simulink model "ESD_Poject_Portable_solar_PV"  (R2024a)
settings: Solver=ode23t  StartTime=0.0  StopTime=5  RelTol=1e-3
undefined symbols (not defined in the file or in its folder): Ion, Lithium
libraries: spsSeriesRLCBranchLib x10, spsCurrentMeasurementLib x4, spsVoltageMeasurementLib x3, spsMosfetLib x2, spsIGBTDiodeLib x2, spsBatteryLib x1, spsDiodeLib x1, spsIGBTLib x1, slpidlib x1, spsPVArrayLib x1, eePwmGenerator x1, spsPWMGeneratorDCDCLib x1
settings Model: Creator=vihan  LastModifiedBy=vihan

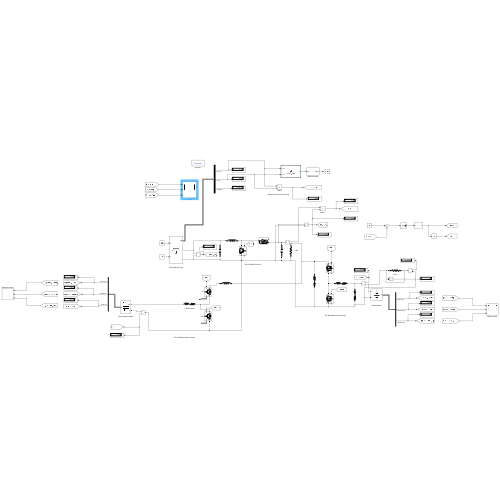
[thumbnail: Simulink's stored preview of the top-level diagram]
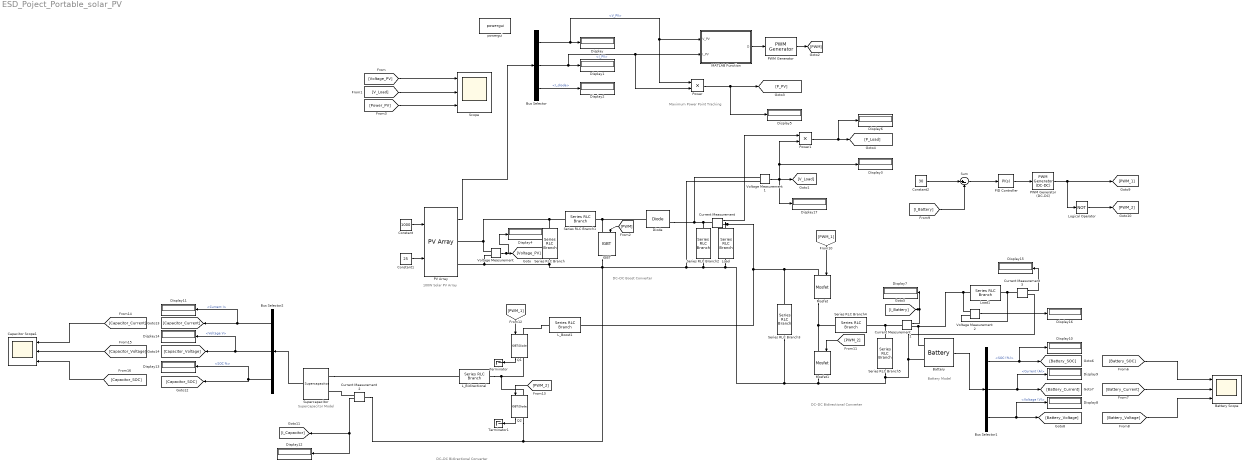
== system ESD_Poject_Portable_solar_PV ==
  note: Supercapacitor Model
  note: Battery Model
  note: DC–DC Bidirectional Converter
  note: Maximum Power Point Tracking
  note: DC–DC Boost Converter
  note: 100W Solar PV Array
  note: DC–DC Bidirectional Converter
  Battery : spsBatteryLib/Battery  BatType=Lithium-Ion  ShowTempParam=off  ThermalPreset=no  ShowAgeParam=off  NomV=7.2  NomQ=5.4  SOC=100  Batt_Tr=30  PresetModel=on  MaxQ=5.4  MinV=5.4  FullV=8.3807  Dis_rate=2.3478  R=0.013333  Normal_OP=4.8835  expZone="[7.7788      0.2653]"  current=[6.5 13 32.5]  Units=Time  Tci=20  NomT=20  T2=-30  MaxQ2=4.8  FullV2=7.1  Normal_OP2=5.655  expZone2="[6.58           1]"  Rca=0.6  ti=2000  Dp=0  Neq0=0  Tsim=1e6  Ta1=25  Qeol=5.4*0.9  Reol=0.013333*1.2  Char_age=[2.3478, 3]  Dis_age=[2.3478, 10]  N1=1500  N2=10500  N3=1000  N4=1400  Ta2=45  N5=950
  Battery Scope : Scope  NumInputPorts=3
  Bus Selector : BusSelector  OutputSignals=V_PV,I_PV,I_diode
  Bus Selector1 : BusSelector  OutputSignals=SOC (%),Current (A),Voltage (V)
  Bus Selector2 : BusSelector  OutputSignals=Current I,Voltage V,SOC %
  Capacitor Scope1 : Scope  NumInputPorts=3
  Constant : Constant  Value=1000
  Constant1 : Constant  Value=25
  Constant2 : Constant  Value=30
  Current Measurement{,1..3} (4 alike) : spsCurrentMeasurementLib/Current Measurement  PhasorSimulation=off  OutputType=Complex  PSBequivalent=0
  Diode : spsDiodeLib/Diode  Ron=0.001  Lon=0  Vf=0.8  IC=0  UseSnubber=0  Rs=500  Cs=250e-9  Measurements=on
  Display{,1..17} (18 alike) : Display
  IGBT : spsIGBTLib/IGBT  Ron=0.001  Lon=0  Vf=1  Tf=1e-6  Tt=2e-6  IC=0  Rs=1e5  Cs=inf  Measurements=on
  L_Bidirectional : spsSeriesRLCBranchLib/Series RLC Branch  LConnTagsString=__new0  RConnTagsString=__new0  BranchType=RL  Resistance=0.05  Inductance=0.355e-3  SetiL0=off  InitialCurrent=0  Capacitance=1e-6  Setx0=off  InitialVoltage=0  Measurements=None
  L_Boost1 : spsSeriesRLCBranchLib/Series RLC Branch  LConnTagsString=__new0  RConnTagsString=__new0  BranchType=L  Resistance=0.05  Inductance=1.5e-3  SetiL0=off  InitialCurrent=0  Capacitance=1e-6  Setx0=off  InitialVoltage=0  Measurements=None
  Load : spsSeriesRLCBranchLib/Series RLC Branch  LConnTagsString=__new0  RConnTagsString=__new0  BranchType=R  Resistance=50  Inductance=1e-3  SetiL0=off  InitialCurrent=0  Capacitance=3000e-6  Setx0=on  InitialVoltage=0  Measurements=None
  Load1 : spsSeriesRLCBranchLib/Series RLC Branch  LConnTagsString=__new0  RConnTagsString=__new0  BranchType=R  Resistance=500000  Inductance=1e-3  SetiL0=off  InitialCurrent=0  Capacitance=3000e-6  Setx0=on  InitialVoltage=0  Measurements=None
  Logical Operator : Logic  Operator=NOT  AllPortsSameDT=off  OutDataTypeStr=boolean
  MATLAB Function : MATLAB Function  TreatAsAtomicUnit=on
  Mosfet : spsMosfetLib/Mosfet  Ron=0.1  Lon=0  Rd=0.01  Vfd=0  IC=0  Rs=1e5  Cs=inf  Measurements=on
  Mosfet1 : spsMosfetLib/Mosfet  Ron=0.1  Lon=0  Rd=0.01  Vfd=0  IC=0  Rs=1e5  Cs=inf  Measurements=on
  PID Controller : slpidlib/PID Controller  Controller=PI  Form=Parallel  TimeDomain=Continuous-time  UseExternalTs=off  SampleTime=-1  IntegratorMethod=Forward Euler  FilterMethod=Forward Euler  ControllerParametersSource=internal  P=1.5  I=25  UseKiTs=off  D=0  UseExternalDerivativeSource=off  N=100  UseFilter=on  TunerSelectOption=Transfer Function Based (PID Tuner App)  InitialConditionSource=internal  InitialConditionForIntegrator=0  InitialConditionForFilter=0  DifferentiatorICPrevScaledInput=0  ExternalReset=none  TrackingMode=off  Kt=1  LimitOutput=on  SatLimitsSource=internal  UpperSaturationLimit=0.95  LowerSaturationLimit=0  LinearizeAsGain=on  AntiWindupMode=none  Kb=1  LimitIntegrator=off  UpperIntegratorSaturationLimit=inf  LowerIntegratorSaturationLimit=-inf  POutMin=[]  POutMax=[]  IOutMin=[]  IOutMax=[]  DOutMin=[]  DOutMax=[]  NOutMin=[]  NOutMax=[]  SumOutMin=[]  SumOutMax=[]  SaturationOutMin=[]  SaturationOutMax=[]  PParamMin=[]  PParamMax=[]  IParamMin=[]  IParamMax=[]  DParamMin=[]  DParamMax=[]  NParamMin=[]  NParamMax=[]  KbParamMin=[]  KbParamMax=[]  KtParamMin=[]  KtParamMax=[]  KbOutMin=[]  KbOutMax=[]  KtOutMin=[]  KtOutMax=[]  IntegratorOutMin=[]  IntegratorOutMax=[]  FilterOutMin=[]  FilterOutMax=[]  SumI1OutMin=[]  SumI1OutMax=[]  SumI2OutMin=[]  SumI2OutMax=[]  SumI3OutMin=[]  SumI3OutMax=[]  SumI4OutMin=[]  SumI4OutMax=[]  SumDOutMin=[]  SumDOutMax=[]  DifferentiatorOutMin=[]  DifferentiatorOutMax=[]  FilterDiffOutCoefMin=[]  FilterDiffOutCoefMax=[]  ReciprocalOutMin=[]  ReciprocalOutMax=[]  SumDenOutMin=[]  SumDenOutMax=[]  SumNumOutMin=[]  SumNumOutMax=[]  DivideOutMin=[]  DivideOutMax=[]  UdiffTsProdOutMin=[]  UdiffTsProdOutMax=[]  NTsProdOutMin=[]  NTsProdOutMax=[]  UintegralTsProdOutMin=[]  UintegralTsProdOutMax=[]  UngainTsProdOutMin=[]  UngainTsProdOutMax=[]  ClampingZeroOutDataTypeStr=Inherit: Inherit via back propagation  ClampingZeroOutMin=[]  ClampingZeroOutMax=[]  FilterDenConstantOutDataTypeStr=Inherit: Inherit via back propagation  FilterDenConstantOutMin=[]  FilterDenConstantOutMax=[]  PCopyOutDataTypeStr=Inherit: Inherit via back propagation  PCopyOutMin=[]  PCopyOutMax=[]  NCopyOutDataTypeStr=Inherit: Inherit via back propagation  NCopyOutMin=[]  NCopyOutMax=[]  IntegratorContinuousStateAttributes=''  IntegratorStateMustResolveToSignalObject=off  IntegratorRTWStateStorageClass=Auto  FilterContinuousStateAttributes=''  FilterStateMustResolveToSignalObject=off  FilterRTWStateStorageClass=Auto  ParallelPVariant=InternalParameters  IdealPVariant=Disabled  IVariant=InternalParameters  DVariant=Disabled  IntegratorVariant=Continuous  SatVariant=Enabled  AWVariant=Passthrough  PCopyVariant=Disabled  TRVariant=Disabled  FdbkBlocksVariant=Forward  IdealPFdbkVariant=Disabled  SatFdbkVariant=Disabled  DerivativeFilterVariant=Disabled  NVariant=Disabled  NCopyVariant=Disabled_SignalSpec  FilterICVariant=Disabled  IntegratorICVariant=InternalICs  ExternalResetVariant=Disabled  TRSumVariant=Passthrough  SumFdbkVariant=Disabled  SumVariant=Sum_PI  TsampFilterVariant=InternalTs  TsampNgainVariant=Passthrough  TsampIntegralVariant=Disabled_SignalSpec  ExternalSaturationOutDataTypeStr=Inherit: Same as second input  DerivativeSourceVariant=Disabled
  PV Array : spsPVArrayLib/PV Array  Npar=1  Nser=1  PlotType=array @ 1000 W/m2 & specified temperatures  S_vec="[ 1000  500  100 ]"  Temp_C_vec="[ 45 25  ]"  ModuleName=User-defined  PlotWhenSelected=off  Pm=100.08  Ncell=36  Voc=21.6  Isc=6  Vm=18  Im=5.56  beta_Voc_pc=-0.36099  alpha_Isc_pc=0.102  beta_Voc=-0.077974  alpha_Isc=0.00612  IL=6.0082  I0=2.2244e-10  nI=0.97355  Rsh=115.4405  Rs=0.15873  RobustModel=off  RobustCellTemperature=313.3991  BAL=on  Tc=1e-6  Tfilter=5e-5
  PWM Generator : eePwmGenerator/PWM Generator  CarrCount=Up  Tper=0.001  Tdelay=0  Ts=5e-5
  PWM Generator (DC-DC) : spsPWMGeneratorDCDCLib/PWM Generator (DC-DC)  Fsw=5000  Ts=1e-6
  Power : Product
  Power1 : Product
  Q1 : spsIGBTDiodeLib/IGBT//Diode  Ron=1e-3  Rs=1e5  Cs=inf  Measurements=on
  Q2 : spsIGBTDiodeLib/IGBT//Diode  Ron=1e-3  Rs=1e5  Cs=inf  Measurements=on
  Scope : Scope  NumInputPorts=3
  Series RLC Branch : spsSeriesRLCBranchLib/Series RLC Branch  LConnTagsString=__new0  RConnTagsString=__new0  BranchType=C  Resistance=1  Inductance=1e-3  SetiL0=off  InitialCurrent=0  Capacitance=1000e-6  Setx0=on  InitialVoltage=0  Measurements=None
  Series RLC Branch1 : spsSeriesRLCBranchLib/Series RLC Branch  LConnTagsString=__new0  RConnTagsString=__new0  BranchType=L  Resistance=1  Inductance=300e-3  SetiL0=on  InitialCurrent=0  Capacitance=1000e-6  Setx0=on  InitialVoltage=0  Measurements=None
  Series RLC Branch2 : spsSeriesRLCBranchLib/Series RLC Branch  LConnTagsString=__new0  RConnTagsString=__new0  BranchType=C  Resistance=1  Inductance=1e-3  SetiL0=off  InitialCurrent=0  Capacitance=3000e-6  Setx0=on  InitialVoltage=0  Measurements=None
  Series RLC Branch3 : spsSeriesRLCBranchLib/Series RLC Branch  LConnTagsString=__new0  RConnTagsString=__new0  BranchType=RC  Resistance=1e-4  Inductance=1e-3  SetiL0=off  InitialCurrent=0  Capacitance=1000e-6  Setx0=off  InitialVoltage=0  Measurements=None
  Series RLC Branch4 : spsSeriesRLCBranchLib/Series RLC Branch  LConnTagsString=__new0  RConnTagsString=__new0  BranchType=RL  Resistance=1e-4  Inductance=13e-3  SetiL0=off  InitialCurrent=0  Capacitance=1000e-6  Setx0=off  InitialVoltage=0  Measurements=None
  Series RLC Branch5 : spsSeriesRLCBranchLib/Series RLC Branch  LConnTagsString=__new0  RConnTagsString=__new0  BranchType=RC  Resistance=1e-4  Inductance=13e-3  SetiL0=off  InitialCurrent=0  Capacitance=20e-6  Setx0=off  InitialVoltage=0  Measurements=None
  Sum : Sum  Inputs=|+-
  Supercapacitor : spsSupercapacitorLib/Supercapacitor  C=10  Rdc=8.9e-3  Voltage=48  Ns=18  Np=1  Vinit=0  Temp=25  PresetModel=off  EstParam=off  Nc=1  r=1e-9  epsilon=6.0208e-10  Ich=10  Vstern="[0.161  2.7  7.8]"  Self_dis=on  Ioc=10  Vself="[48  47.8  47.06  44.65]"  demandeplot=off  I="[10  20 100  500]"  Units=sec  Vmax=0  If=0  deltaV=0  alpha=0  sec=0
      settings: LibrarySourceBlock=sps_lib/Sources/Supercapacitor
  Terminator : Terminator
  Terminator1 : Terminator
  Voltage Measurement : spsVoltageMeasurementLib/Voltage Measurement  PhasorSimulation=off  OutputType=Complex  PSBequivalent=0
  Voltage Measurement1 : spsVoltageMeasurementLib/Voltage Measurement  PhasorSimulation=off  OutputType=Complex  PSBequivalent=0
  Voltage Measurement2 : spsVoltageMeasurementLib/Voltage Measurement  PhasorSimulation=off  OutputType=Complex  PSBequivalent=0
  powergui : sps_lib/powergui  Priority=1  SimulationMode=Continuous  SampleTime=50e-6  frequency=60  Iterations=50  frequencyindice=0  Pbase=100e6  ErrMax=1e-4  UnitsV=kV  UnitsW=MW  buscounter=0  FunctionMessages=off  echomessages=off  EnableUseOfTLC=off  CurrentSourceSwitches=off  DisableSnubberDevices=off  DisableRonSwitches=off  DisableVfSwitches=off  DisplayEquations=off  AutomaticDiscreteSolvers=off  SolverType=Tustin/Backward Euler (TBE)  Interpol=off  ExternalGateDelay=off  methode=off  Ts=100  x0status=blocks  SPID=on  SwTol=0  HookPort=off  NonlinearTolerance=1e-4  nMaxIteration=100  ContinueOnMaxIteration=off  RestoreLinks=warning  ResistiveCurrentMeasurement=off  Frange=[0:2:500]  Ylog=off  Xlog=on  ShowGrid=off  save=off  variable=ZData  structure=0  ZoomFFT=off  StartTime=0.0  cycles=1  DisplayStyle=1  fundamental=60  FreqAxis=off  MaxFrequency=1000  frequencyindicesteady=1  RmsSteady=1  display=off
  wires:
  Constant1/1 -> PV Array/2
  Constant/1 -> PV Array/1
  PV Array/1 -> Bus Selector/1
  Bus Selector/1 -> Power/1, MATLAB Function/1(V_PV), Display/1  "<V_PV>"
  Bus Selector/2 -> Power/2, MATLAB Function/2(I_PV), Display1/1  "<I_PV>"
  Bus Selector/3 -> Display2/1  "<I_diode>"
  Voltage Measurement/1 -> Display4/1, [Voltage_PV]
  [Voltage_PV] -> Scope/1
  [V_Load] -> Scope/2
  MATLAB Function/1(D) -> PWM Generator/1
  PWM Generator/1 -> [PWM]
  [PWM] -> IGBT/1
  Power/1 -> Display5/1, [P_PV]
  [Power_PV] -> Scope/3
  Power1/1 -> Display6/1, [P_Load]
  Voltage Measurement1/1 -> Display17/1, [V_Load], Power1/2, Display3/1
  Current Measurement/1 -> Power1/1
  Battery/1 -> Bus Selector1/1
  Current Measurement1/1 -> [I_Battery], Display7/1
  Bus Selector1/1 -> Display10/1, [Battery_SOC]  "<SOC (%)>"
  Bus Selector1/2 -> Display9/1, [Battery_Current]  "<Current (A)>"
  Bus Selector1/3 -> Display8/1, [Battery_Voltage]  "<Voltage (V)>"
  [Battery_Current] -> Battery Scope/2
  [Battery_SOC] -> Battery Scope/1
  [Battery_Voltage] -> Battery Scope/3
  [I_Battery] -> Sum/2
  Sum/1 -> PID Controller/1
  PID Controller/1 -> PWM Generator (DC-DC)/1
  PWM Generator (DC-DC)/1 -> [PWM_1], Logical Operator/1
  Logical Operator/1 -> [PWM_2]
  [PWM_1] -> Mosfet/1
  [PWM_2] -> Mosfet1/1
  Constant2/1 -> Sum/1
  Bus Selector2/2 -> [Capacitor_Voltage], Display14/1  "<Voltage V>"
  Bus Selector2/1 -> [Capacitor_Current], Display11/1  "<Current I>"
  Bus Selector2/3 -> [Capacitor_SOC], Display13/1  "<SOC %>"
  Current Measurement2/1 -> [I_Capacitor], Display12/1
  [Capacitor_Voltage] -> Capacitor Scope1/2
  [Capacitor_Current] -> Capacitor Scope1/1
  [Capacitor_SOC] -> Capacitor Scope1/3
  Supercapacitor/1 -> Bus Selector2/1
  Q1/1 -> Terminator/1
  Q2/1 -> Terminator1/1
  [PWM_2] -> Q2/1
  [PWM_1] -> Q1/1
  Current Measurement3/1 -> Display15/1
  Voltage Measurement2/1 -> Display16/1
  connections:
  Series RLC Branch/LConn1 -- Voltage Measurement/LConn1 -- PV Array/RConn1 -- Series RLC Branch1/LConn1
  Series RLC Branch1/RConn1 -- Diode/LConn1 -- IGBT/LConn1
  Diode/RConn1 -- Voltage Measurement1/LConn1 -- Current Measurement/LConn1 -- Series RLC Branch2/LConn1
  Mosfet/RConn1 -- Series RLC Branch4/RConn1 -- Mosfet1/LConn1
  Series RLC Branch5/RConn1 -- Current Measurement1/LConn1 -- Series RLC Branch4/LConn1
  Load1/LConn1 -- Voltage Measurement2/LConn1 -- Battery/LConn1 -- Current Measurement1/RConn1
  Mosfet/LConn1 -- Load/RConn1 -- Current Measurement/RConn1 -- L_Boost1/LConn1 -- Series RLC Branch3/LConn1
  Current Measurement2/RConn1 -- Supercapacitor/LConn2
  Supercapacitor/LConn1 -- L_Bidirectional/RConn1
  Battery/LConn2 -- Current Measurement3/RConn1 -- Series RLC Branch5/LConn1 -- Mosfet1/RConn1 -- Voltage Measurement1/LConn2 -- IGBT/RConn1 -- Current Measurement2/LConn1 -- Q2/RConn1 -- Series RLC Branch/RConn1 -- Voltage Measurement/LConn2 -- PV Array/RConn2 -- Series RLC Branch2/RConn1 -- Load/LConn1 -- Series RLC Branch3/RConn1
  Q1/RConn1 -- L_Bidirectional/LConn1 -- Q2/LConn1
  L_Boost1/RConn1 -- Q1/LConn1
  Current Measurement3/LConn1 -- Voltage Measurement2/LConn2 -- Load1/RConn1

== matlab function ESD_Poject_Portable_solar_PV/MATLAB Function ==
  settings: updateMethod=DISCRETE
  data: V_PV input; D output; I_PV input
function D = MPPT_PO(V_PV, I_PV)

% Persistent variables to store previous values
persistent D_prev P_prev V_prev

% Initialization of persistent variables
if isempty(D_prev)
    D_prev = 0.5; % Initial duty ratio (50%)
    P_prev = 0;
    V_prev = 0;
end

% Step size for duty adjustment
deltaD = 0.01;

% Calculate present PV power
P = V_PV * I_PV;

% Perturb & Observe logic
if (P > P_prev)
    if (V_PV > V_prev)
        D = D_prev + deltaD;
    else
        D = D_prev - deltaD;
    end
else
    if (V_PV > V_prev)
        D = D_prev - deltaD;
    else
        D = D_prev + deltaD;
    end
end

% Duty cycle limits
D = max(min(D, 1), 0);

% Update stored values
D_prev = D;
P_prev = P;
V_prev = V_PV;
